simulink subsystem "deadReckoning"  (R2026a)
settings: Solver=VariableStepAuto
values from neighbouring files (symbols this model uses):
  navControl = 1    [navParams.sldd]
libraries: aerolibutil x1, sharedutil x1
settings Model: Creator=maxhu  LastModifiedBy=maxhu

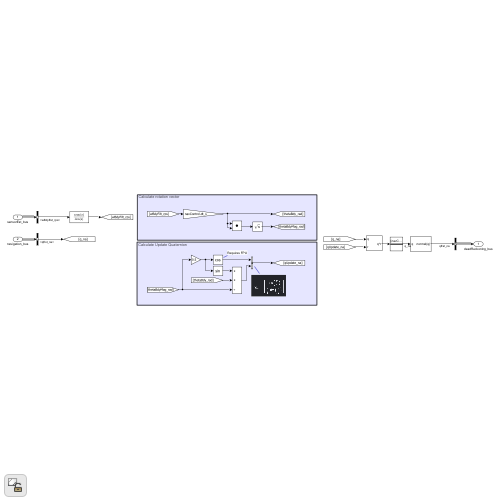
[thumbnail: Simulink's stored preview of the top-level diagram]
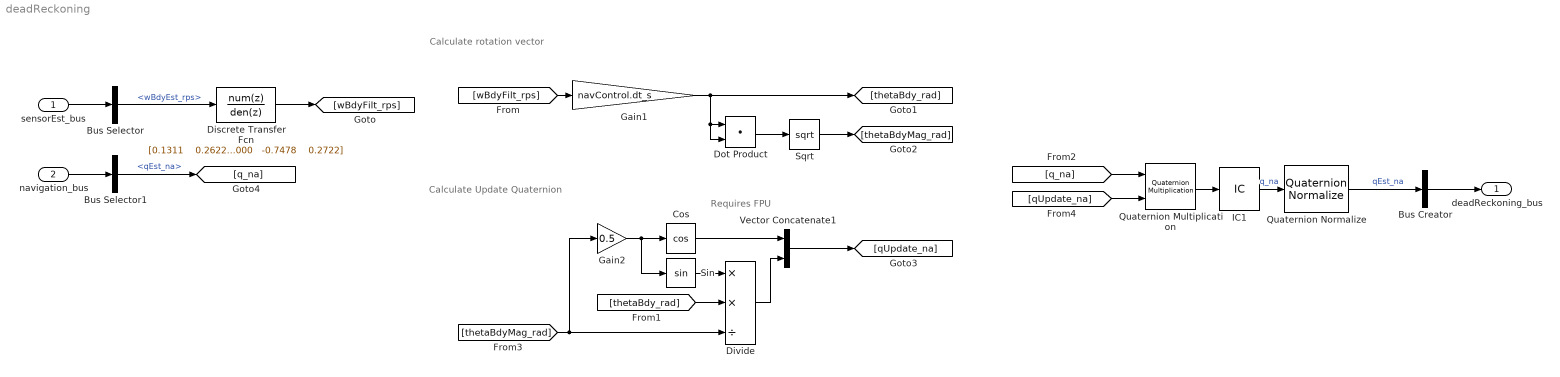
== system deadReckoning ==
  note: Calculate Update Quaternion
  note: Calculate rotation vector
  note: Requires FPU
  sensorEst_bus : Inport
  navigation_bus : Inport  Port=2
  Bus Creator : BusCreator  Inputs=1
  Bus Selector : BusSelector  OutputSignals=wBdyEst_rps
  Bus Selector1 : BusSelector  OutputSignals=qEst_na
  Cos : Trigonometry  Operator=cos
  Discrete Transfer Fcn : DiscreteTransferFcn  Numerator="[0.1311    0.2622    0.1311]"  Denominator="[1.0000   -0.7478    0.2722]"
  Divide : Product  Inputs=**/
  Dot Product : DotProduct  OutDataTypeStr=Inherit: Inherit via internal rule
  Gain1 : Gain  Gain=navControl.dt_s
  Gain2 : Gain  Gain=0.5
  IC1 : InitialCondition  Value=navControl.q0_na
  Quaternion Multiplication : aerolibutil/Quaternion Multiplication
  Quaternion Normalize : sharedutil/Quaternion Normalize  aMode=aMode
  Sin : Trigonometry
  Sqrt : Sqrt
  Vector Concatenate1 : Concatenate
  deadReckoning_bus : Outport
  wires:
  sensorEst_bus/1 -> Bus Selector/1
  [wBdyFilt_rps] -> Gain1/1
  Dot Product/1 -> Sqrt/1
  Gain1/1 -> [thetaBdy_rad], Dot Product/1, Dot Product/2
  Sqrt/1 -> [thetaBdyMag_rad]
  Gain2/1 -> Cos/1, Sin/1
  [thetaBdyMag_rad] -> Divide/3, Gain2/1
  Sin/1 -> Divide/1
  Cos/1 -> Vector Concatenate1/1
  Divide/1 -> Vector Concatenate1/2
  Vector Concatenate1/1 -> [qUpdate_na]
  [q_na] -> Quaternion Multiplication/1
  [qUpdate_na] -> Quaternion Multiplication/2
  Quaternion Multiplication/1 -> IC1/1
  [thetaBdy_rad] -> Divide/2
  navigation_bus/1 -> Bus Selector1/1
  Bus Selector1/1 -> [q_na]  "<qEst_na>"
  Bus Selector/1 -> Discrete Transfer Fcn/1  "<wBdyEst_rps>"
  Discrete Transfer Fcn/1 -> [wBdyFilt_rps]
  Quaternion Normalize/1 -> Bus Creator/1  "qEst_na"
  IC1/1 -> Quaternion Normalize/1  "q_na"
  Bus Creator/1 -> deadReckoning_bus/1
